simulink model "Experimento1"  (R2019a)
settings: Solver=FixedStepAuto  StartTime=0.0  StopTime=1e-4  FixedStep=1e-7  RelTol=1e-3
libraries: simulink x1
settings Model: Creator=marco  LastModifiedBy=marco

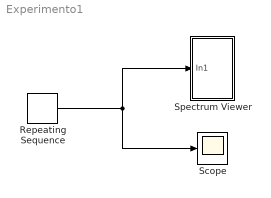
== system Experimento1 ==
  Repeating Sequence : simulink/Sources/Repeating Sequence  rep_seq_t=[0 0.5e-5 1e-5]  rep_seq_y=[0 0.1 0]
  Scope : Scope
  Spectrum Viewer : Subsystem
  wires:
  Repeating Sequence/1 -> Spectrum Viewer/1(In1), Scope/1

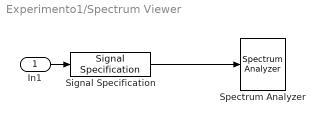
== system Experimento1/Spectrum Viewer ==
  In1 : Inport
  Signal Specification : SignalSpecification  SampleTime=1e-6
  Spectrum Analyzer : SpectrumAnalyzer
  wires:
  Signal Specification/1 -> Spectrum Analyzer/1
  In1/1 -> Signal Specification/1
